simulink model "ROBUST_ROLL_OVER"  (R2023a)
settings: Solver=VariableStepAuto  StartTime=0.0  StopTime=6  RelTol=1e-3
values from neighbouring files (symbols this model uses):
  C = eye(4)    [CONTROL_ROLL_OVER.m]    (also in Modelo_roll_control.m; State_space_robust.m)
  D = zeros(4,1)    [CONTROL_ROLL_OVER.m]    (also in Modelo_roll_control.m = zeros(1,4); State_space_robust.m = zeros(1,4))
  k = H_inf_robust(A1,A2,A3,A4,B1,B2,B3,B4,W1,W2,W3,W4,C1,D12,D11)    [CONTROL_ROLL_OVER.m]    (also in Modelo_roll_control.m; State_space_robust.m)
undefined symbols (not defined in the file or in its folder): sigbuilder_block
settings Model: Creator=csanc  LastModifiedBy=csanc

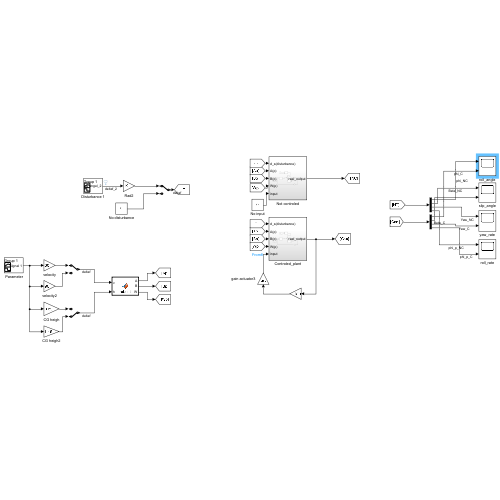
[thumbnail: Simulink's stored preview of the top-level diagram]
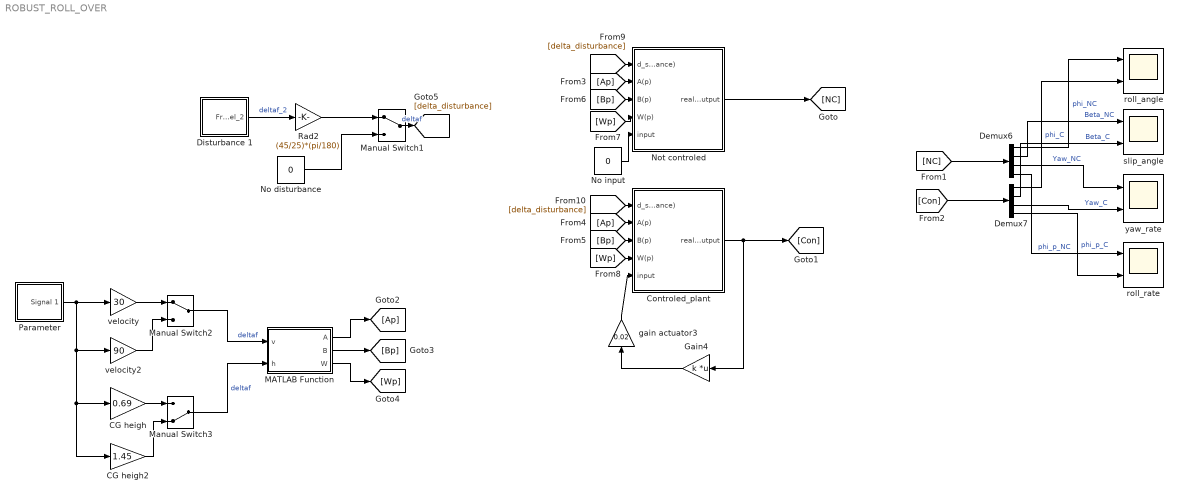
== system ROBUST_ROLL_OVER ==
  " Parameter" : Subsystem  Tag=STV Subsys  LoadFcn=sigbuilder_block('load');  StartFcn=sigbuilder_block('start');  StopFcn=sigbuilder_block('stop');  ClipboardFcn=sigbuilder_block('clipboard');  mask(Sigbuilder block){tuvar=[0:10]}
      mask help: Simulink:masks:SigbuilderBlock_MD
      mask init:
      | if ~strcmp(get_param(bdroot(gcbh),'SimulationStatus'),'stopped') tuvar = sigbuilder_block('maskInit'); end
      settings: CopyFcn=sigbuilder_block('copy');  DeleteFcn=sigbuilder_block('delete');  ModelCloseFcn=sigbuilder_block('modelClose');  PreSaveFcn=sigbuilder_block('preSave');  PauseFcn=sigbuilder_block('pause');  ContinueFcn=sigbuilder_block('continue');  NameChangeFcn=sigbuilder_block('namechange');  OpenFcn=sigbuilder_block('open',[265.8 141.6 550.8 400.2 ]);  CloseFcn=sigbuilder_block('close');
      mask Display: plot(0, 0, 100, 100,[2, 2, 32, 32, 2], [68, 8, 8, 68, 68],[32, 2], [38, 38], [32, 19, 2],[53, 60, 44], [32, 17, 17, 2],[16, 16, 31, 31]);txt = getActiveGroup(gcbh);text(2, 100, txt,'verticalAlignment', 'top');
  CG heigh : Gain  Gain=0.69
  CG heigh2 : Gain  Gain=1.45
  Controled_plant : Subsystem
  Demux6 : Demux
  Demux7 : Demux
  Disturbance 1 : Subsystem  Tag=STV Subsys  LoadFcn=sigbuilder_block('load');  StartFcn=sigbuilder_block('start');  StopFcn=sigbuilder_block('stop');  ClipboardFcn=sigbuilder_block('clipboard');  mask(Sigbuilder block){tuvar=[0:10]}
      mask help: Simulink:masks:SigbuilderBlock_MD
      mask init:
      | if ~strcmp(get_param(bdroot(gcbh),'SimulationStatus'),'stopped') tuvar = sigbuilder_block('maskInit'); end
      settings: CopyFcn=sigbuilder_block('copy');  DeleteFcn=sigbuilder_block('delete');  ModelCloseFcn=sigbuilder_block('modelClose');  PreSaveFcn=sigbuilder_block('preSave');  PauseFcn=sigbuilder_block('pause');  ContinueFcn=sigbuilder_block('continue');  NameChangeFcn=sigbuilder_block('namechange');  OpenFcn=sigbuilder_block('open',[265.8 141.6 550.8 400.2 ]);  CloseFcn=sigbuilder_block('close');
      mask Display: plot(0, 0, 100, 100,[2, 2, 32, 32, 2], [68, 8, 8, 68, 68],[32, 2], [38, 38], [32, 19, 2],[53, 60, 44], [32, 17, 17, 2],[16, 16, 31, 31]);txt = getActiveGroup(gcbh);text(2, 100, txt,'verticalAlignment', 'top');
  Gain4 : Gain  Gain=k  Multiplication=Matrix(K*u)
  MATLAB Function : MATLAB Function  TreatAsAtomicUnit=on
  Manual Switch1 : ManualSwitch
  Manual Switch2 : ManualSwitch
  Manual Switch3 : ManualSwitch  CurrentSetting=0
  No disturbance : Constant  Value=0
  No input : Constant  Value=0
  Not controled : Subsystem
  Rad2 : Gain  Gain=(45/25)*(pi/180)
  gain actuator3 : Gain  Gain=0.02
  roll_angle : Scope  NumInputPorts=2
  roll_rate : Scope  NumInputPorts=2
  slip_angle : Scope  NumInputPorts=2
  velocity : Gain  Gain=30
  velocity2 : Gain  Gain=90
  yaw_rate : Scope  NumInputPorts=2
  wires:
  Manual Switch3/1 -> MATLAB Function/2(h)  "deltaf"
  Manual Switch2/1 -> MATLAB Function/1(v)  "deltaf"
  CG heigh2/1 -> Manual Switch3/2
  CG heigh/1 -> Manual Switch3/1
  No disturbance/1 -> Manual Switch1/2
  Rad2/1 -> Manual Switch1/1
  " Parameter"/1(Signal 1) -> velocity2/1, CG heigh2/1, CG heigh/1, velocity/1
  Disturbance 1/1(Front steering angel_2) -> Rad2/1  "deltaf_2"
  velocity2/1 -> Manual Switch2/2
  velocity/1 -> Manual Switch2/1
  Gain4/1 -> gain actuator3/1
  Controled_plant/1(real_output) -> [Con], Gain4/1
  gain actuator3/1 -> Controled_plant/5(input)
  Demux6/4 -> roll_rate/1  "phi_p_NC"
  Demux7/1 -> roll_angle/2  "phi_C"
  Demux7/2 -> slip_angle/2  "Beta_C"
  Demux7/3 -> yaw_rate/2  "Yaw_C"
  Demux7/4 -> roll_rate/2  "phi_p_C"
  Demux6/3 -> yaw_rate/1  "Yaw_NC"
  [Con] -> Demux7/1
  Demux6/2 -> slip_angle/1  "Beta_NC"
  [NC] -> Demux6/1
  Demux6/1 -> roll_angle/1  "phi_NC"
  Not controled/1(real_output) -> [NC]
  No input/1 -> Not controled/5(input)
  MATLAB Function/1(A) -> [Ap]
  [Ap] -> Not controled/2(A(p))
  [Ap] -> Controled_plant/2(A(p))
  MATLAB Function/2(B) -> [Bp]
  [Bp] -> Not controled/3(B(p))
  [Bp] -> Controled_plant/3(B(p))
  MATLAB Function/3(W) -> [Wp]
  [Wp] -> Not controled/4(W(p))
  [Wp] -> Controled_plant/4(W(p))
  Manual Switch1/1 -> [delta_disturbance]  "deltaf"
  [delta_disturbance] -> Controled_plant/1(d_s(disturbance))
  [delta_disturbance] -> Not controled/1(d_s(disturbance))

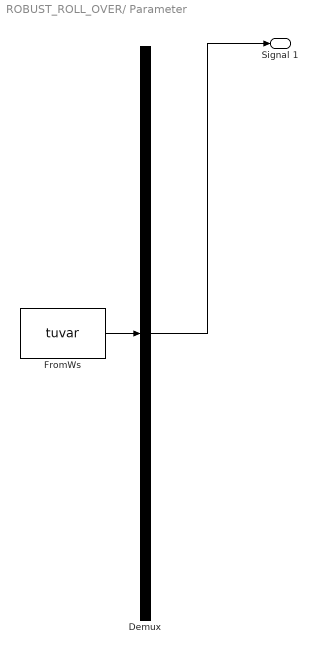
== system ROBUST_ROLL_OVER/ Parameter ==
  Demux : Demux  Tag=STV Demux  Outputs=1
      settings: DisplayOption=none
  FromWs : FromWorkspace  Tag=STV FromWs  VariableName=tuvar
      SigBuilderData=|
      | common.afterFinalStr = 'Extrapolate'
      | common.sampleTime = 0
      | dataSet.timeRange = [0 3]
      | dataSet.name = 'Group 1'
      | sbobj.Groups.Name = 'Group 1'
      | sbobj.Groups.Signals.Name = 'Signal 1'
      | sbobj.Groups.Signals.XData = [0 3]
      | sbobj.Groups.Signals.YData = [1 1]
      | sbobj.Groups.TimeRange = [0 3]
  Signal 1 : Outport  Tag=STV Outport
  wires:
  FromWs/1 -> Demux/1
  Demux/1 -> Signal 1/1

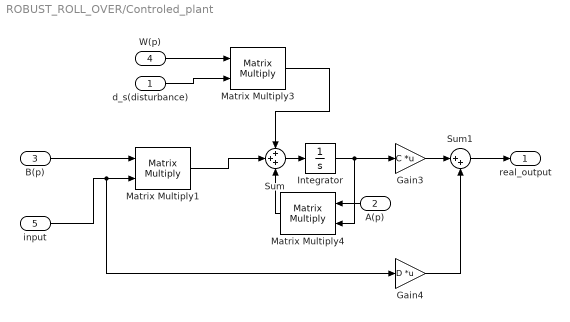
== system ROBUST_ROLL_OVER/Controled_plant ==
  d_s(disturbance) : Inport
  A(p) : Inport  Port=2
  B(p) : Inport  Port=3
  W(p) : Inport  Port=4
  input : Inport  Port=5
  Gain3 : Gain  Gain=C  Multiplication=Matrix(K*u)
  Gain4 : Gain  Gain=D  Multiplication=Matrix(K*u)
  Integrator : Integrator  InitialCondition=[0, 0, 0, 0]
  Matrix Multiply1 : Product  Multiplication=Matrix(*)
  Matrix Multiply3 : Product  Multiplication=Matrix(*)
  Matrix Multiply4 : Product  Multiplication=Matrix(*)
  Sum : Sum  Inputs=+++
  Sum1 : Sum  Inputs=|++
  real_output : Outport
  wires:
  Integrator/1 -> Matrix Multiply4/2, Gain3/1
  Matrix Multiply4/1 -> Sum/3
  Gain3/1 -> Sum1/1
  A(p)/1 -> Matrix Multiply4/1
  Sum1/1 -> real_output/1
  Gain4/1 -> Sum1/2
  Sum/1 -> Integrator/1
  Matrix Multiply3/1 -> Sum/1
  d_s(disturbance)/1 -> Matrix Multiply3/2
  W(p)/1 -> Matrix Multiply3/1
  B(p)/1 -> Matrix Multiply1/1
  input/1 -> Gain4/1, Matrix Multiply1/2
  Matrix Multiply1/1 -> Sum/2

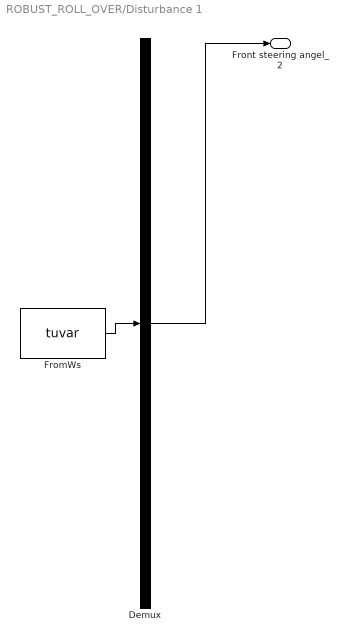
== system ROBUST_ROLL_OVER/Disturbance 1 ==
  Demux : Demux  Tag=STV Demux  Outputs=1
      settings: DisplayOption=none
  FromWs : FromWorkspace  Tag=STV FromWs  VariableName=tuvar
      SigBuilderData=|
      | common.afterFinalStr = 'Extrapolate'
      | common.sampleTime = 0
      | dataSet.timeRange = [0 3]
      | dataSet.name = 'Group 1'
      | sbobj.Groups.Name = 'Group 1'
      | sbobj.Groups.Signals.Name = 'Front steering angel_2'
      | sbobj.Groups.Signals.XData = [0 0.187490625469 0.374981250937 0.562471876406 0.749962501875 0.937453127344 1.12494375281 1.31243437828 1.49992500375 1.68741562922 1.87490625469 2.06239688016 2.24988750562 2.43737813109 2.62486875656 2.81235938203 2.9998500075 3]
      | sbobj.Groups.Signals.YData = [0 0.565685424949 0.8 0.565685424949 9.79717439318e-17 -0.565685424949 -0.8 -0.565685424949 0 0 0 0 0 0 0 0 0 0]
      | sbobj.Groups.TimeRange = [0 3]
  Front steering angel_2 : Outport  Tag=STV Outport
  wires:
  FromWs/1 -> Demux/1
  Demux/1 -> Front steering angel_2/1

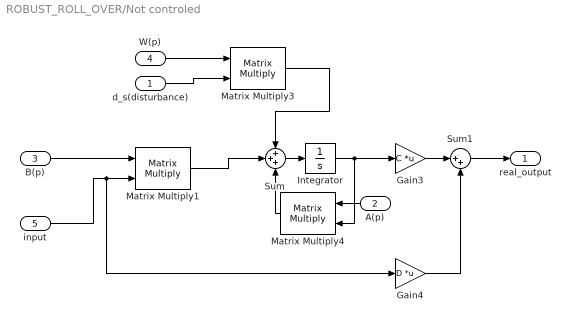
== system ROBUST_ROLL_OVER/Not controled ==
  d_s(disturbance) : Inport
  A(p) : Inport  Port=2
  B(p) : Inport  Port=3
  W(p) : Inport  Port=4
  input : Inport  Port=5
  Gain3 : Gain  Gain=C  Multiplication=Matrix(K*u)
  Gain4 : Gain  Gain=D  Multiplication=Matrix(K*u)
  Integrator : Integrator  InitialCondition=[0, 0, 0, 0]
  Matrix Multiply1 : Product  Multiplication=Matrix(*)
  Matrix Multiply3 : Product  Multiplication=Matrix(*)
  Matrix Multiply4 : Product  Multiplication=Matrix(*)
  Sum : Sum  Inputs=+++
  Sum1 : Sum  Inputs=|++
  real_output : Outport
  wires:
  Integrator/1 -> Matrix Multiply4/2, Gain3/1
  Matrix Multiply4/1 -> Sum/3
  Gain3/1 -> Sum1/1
  A(p)/1 -> Matrix Multiply4/1
  Sum1/1 -> real_output/1
  Gain4/1 -> Sum1/2
  Sum/1 -> Integrator/1
  Matrix Multiply3/1 -> Sum/1
  d_s(disturbance)/1 -> Matrix Multiply3/2
  W(p)/1 -> Matrix Multiply3/1
  B(p)/1 -> Matrix Multiply1/1
  input/1 -> Gain4/1, Matrix Multiply1/2
  Matrix Multiply1/1 -> Sum/2

== matlab function ROBUST_ROLL_OVER/MATLAB Function ==
  data: v input; A output; h input; B output; W output
function  [A,B,W]  = robust(v,h)
%% Data...................................................................
m=14300;
m2=12487;
cf=582000;
cr=783000;
mu=1;
lf=1.95;
lr=1.54;
Jz=34917;
J2x=24201;
g=9.81;
dfip=100000;
cfi=457000;
T=1.99;
hr=0.68;
Ifi=J2x+(m2*(h^2));%
Yb=(cf+cr)*mu;%
Nb=((cf*lf)+(cr*lr))*mu;%
Nr=((cf*(lf^2))+(cr*(lr^2)))*mu;%
sigma=(m2*g*h)-cfi;%

%% Matrici del sistema


%% ...............State Space Representation...............................
E=[1,0,0,0;0,m,0,-h*m2;0,0,Jz,0;0,h*m2,0,Ifi];
E1=inv(E);
F=[0,0,0,1;0,-Yb/v,-((Nb/v)-(m*v)),0;0,-Nb/v,-Nr/v,0;sigma,0,m2*h*v,-dfip];
A=E1*F;


G=[0;cf*mu;cf*lf*mu;0];
B=E1*G;
%b11=B(1,1);
%b21=B(2,1);
%b31=B(3,1);
%b41=B(4,1);
%B = [b11 b21 b31 b41]

W=B

end
